simulink model "Lidar_System_FullState_Apr19_2015_Triangle"  (Simulink 7.3)
settings: Solver=FixedStepDiscrete  StartTime=0.0  StopTime=inf  FixedStep=0.1  MaxStep=0.2  RelTol=1e-3
undefined symbols (not defined in the file): strel
libraries: dspmtrx3 x9, simulink x7, vipstatistics x3, vipmorphops x3, dspstat3 x3, dspindex x1
(part 1 of 2)
settings Model: Creator=gclayton  LastModifiedBy=wildcat
settings DebuggingCC: InheritedTsInSrcMsg=none
settings RTWCC: SystemTargetFile=rlnx.tlc  GenCodeOnly=on  TemplateMakefile=rlnx_ubuntu.tmf  Description=Linux Real-Time Target  ProcessScript=rlnx_make_rtw_hook
settings RTWCC: CustomInclude=|
  | /usr/local/include/opencv/
  | /usr/local/include/
settings CodeAppCC: GenerateComments=off  SimulinkBlockComments=off
settings STFCustomTargetCC: ModelReferenceCompliant=off  MatFileLogging=on  SystemTargetFile=rlnx.tlc
settings GRTTargetCC: ModelReferenceCompliant=off  ParMdlRefBuildCompliant=off  CompOptLevelCompliant=off
settings CustomProperty: DataType=string  Value="-lm -ldl /usr/local/lib/libopencv_highgui.so.2.4 /usr/local/lib/libopencv_core.so.2.4 /usr/local/lib/libopencv_imgproc.so.2.4  -lc_urg -lc_urg_connection -lc_urg_system -lphidget21 -llcm"
settings EnumStrPairs: String=PC

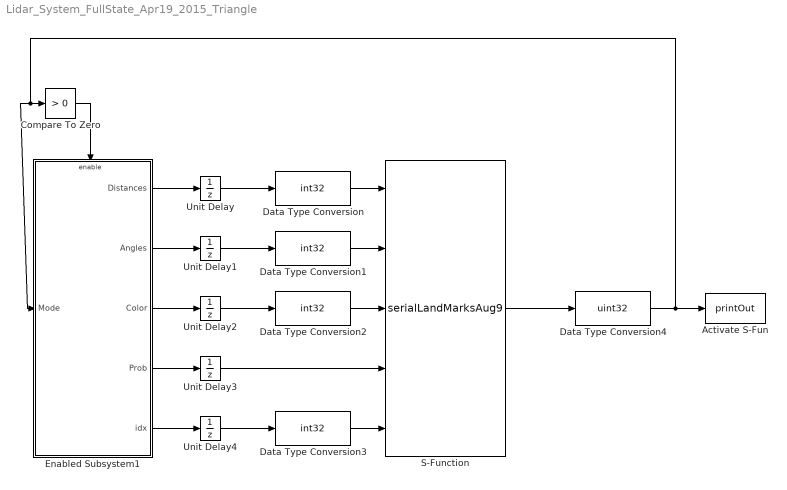
== system Lidar_System_FullState_Apr19_2015_Triangle ==
  Activate S-Fun : S-Function  FunctionName=printOut  EnableBusSupport=off
  Compare To Zero : simulink/Logic and Bit Operations/Compare To Zero  SystemSampleTime=-1  relop=>  LogicOutDataTypeMode=uint8  ZeroCross=off
  Data Type Conversion{,1..3} (4 alike) : DataTypeConversion  OutDataTypeMode=int32  OutDataType=fixdt(1, 16)  OutScaling=2^0  OutDataTypeStr=int32
  Data Type Conversion4 : DataTypeConversion  OutDataTypeMode=uint32  OutDataType=fixdt(1, 16)  OutScaling=2^0  OutDataTypeStr=uint32
  Enabled Subsystem1 : Subsystem  TreatAsAtomicUnit=on
  S-Function : S-Function  FunctionName=serialLandMarksAug9  EnableBusSupport=off
  Unit Delay : UnitDelay  X0=zeros(1,12)  SampleTime=-1
  Unit Delay1 : UnitDelay  X0=zeros(1,12)  SampleTime=-1
  Unit Delay2 : UnitDelay  X0=zeros(4,1)  SampleTime=-1
  Unit Delay3 : UnitDelay  X0=zeros(4,1)  SampleTime=-1
  Unit Delay4 : UnitDelay  X0=zeros(4,1)  SampleTime=-1
  wires:
  Compare To Zero/1 -> Enabled Subsystem1/Enable
  Data Type Conversion4/1 -> Activate S-Fun/1, Compare To Zero/1, Enabled Subsystem1/1(Mode)
  S-Function/1 -> Data Type Conversion4/1
  Enabled Subsystem1/2(Angles) -> Unit Delay1/1
  Enabled Subsystem1/1(Distances) -> Unit Delay/1
  Enabled Subsystem1/3(Color) -> Unit Delay2/1
  Enabled Subsystem1/4(Prob) -> Unit Delay3/1
  Enabled Subsystem1/5(idx) -> Unit Delay4/1
  Unit Delay/1 -> Data Type Conversion/1
  Unit Delay1/1 -> Data Type Conversion1/1
  Unit Delay2/1 -> Data Type Conversion2/1
  Unit Delay4/1 -> Data Type Conversion3/1
  Data Type Conversion/1 -> S-Function/1
  Data Type Conversion1/1 -> S-Function/2
  Data Type Conversion2/1 -> S-Function/3
  Unit Delay3/1 -> S-Function/4
  Data Type Conversion3/1 -> S-Function/5

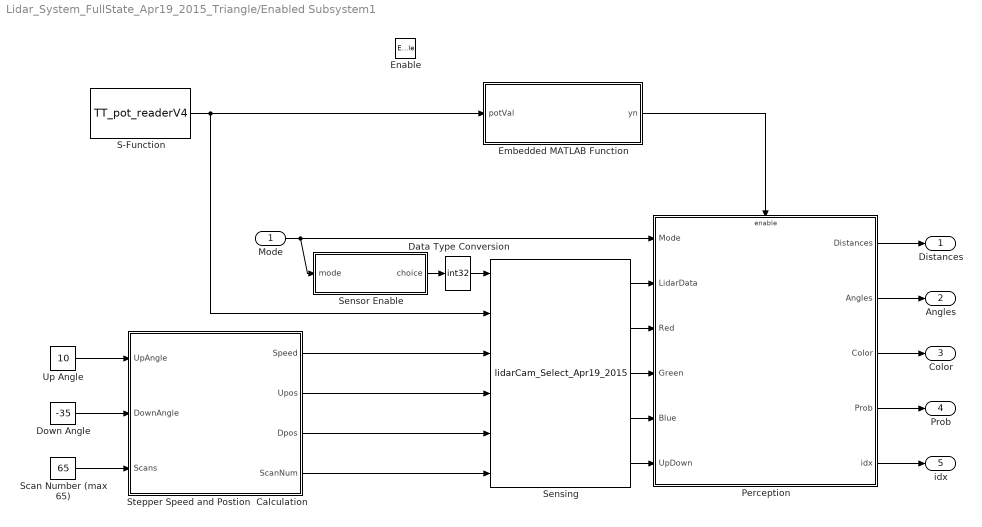
== system Lidar_System_FullState_Apr19_2015_Triangle/Enabled Subsystem1 ==
  Mode : Inport  OutDataType=fixdt(1, 16)  OutScaling=2^0
  Enable : EnablePort
  Data Type Conversion : DataTypeConversion  OutDataTypeMode=int32  OutDataType=fixdt(1, 16)  OutScaling=2^0  OutDataTypeStr=int32
  Down Angle : Constant  Value=-35  OutDataType=fixdt(1, 16)  OutScaling=2^0
  Embedded MATLAB Function : Stateflow chart
  Perception : Subsystem  TreatAsAtomicUnit=on
  S-Function : S-Function  FunctionName=TT_pot_readerV4  EnableBusSupport=off
  Scan Number (max 65) : Constant  Value=65  OutDataType=fixdt(1, 16)  OutScaling=2^0
  Sensing : S-Function  FunctionName=lidarCam_Select_Apr19_2015  EnableBusSupport=off
  Sensor Enable : Stateflow chart
  Stepper Speed and Postion  Calculation : Stateflow chart
  Up Angle : Constant  Value=10  OutDataType=fixdt(1, 16)  OutScaling=2^0
  Distances : Outport  OutDataType=fixdt(1, 16)  OutScaling=2^0
  Angles : Outport  Port=2  OutDataType=fixdt(1, 16)  OutScaling=2^0
  Color : Outport  Port=3  OutDataType=fixdt(1, 16)  OutScaling=2^0
  Prob : Outport  Port=4  OutDataType=fixdt(1, 16)  OutScaling=2^0
  idx : Outport  Port=5  OutDataType=fixdt(1, 16)  OutScaling=2^0
  wires:
  Embedded MATLAB Function/1(yn) -> Perception/Enable
  Sensing/1 -> Perception/2(LidarData)
  Sensing/5 -> Perception/6(UpDown)
  Sensing/2 -> Perception/3(Red)
  Sensing/3 -> Perception/4(Green)
  Sensing/4 -> Perception/5(Blue)
  Mode/1 -> Perception/1(Mode), Sensor Enable/1(mode)
  Down Angle/1 -> Stepper Speed and Postion  Calculation/2(DownAngle)
  Up Angle/1 -> Stepper Speed and Postion  Calculation/1(UpAngle)
  Scan Number (max 65)/1 -> Stepper Speed and Postion  Calculation/3(Scans)
  Stepper Speed and Postion  Calculation/1(Speed) -> Sensing/3
  Stepper Speed and Postion  Calculation/2(Upos) -> Sensing/4
  Stepper Speed and Postion  Calculation/3(Dpos) -> Sensing/5
  Stepper Speed and Postion  Calculation/4(ScanNum) -> Sensing/6
  S-Function/1 -> Embedded MATLAB Function/1(potVal), Sensing/2
  Sensor Enable/1(choice) -> Data Type Conversion/1
  Data Type Conversion/1 -> Sensing/1
  Perception/1(Distances) -> Distances/1
  Perception/2(Angles) -> Angles/1
  Perception/3(Color) -> Color/1
  Perception/4(Prob) -> Prob/1
  Perception/5(idx) -> idx/1

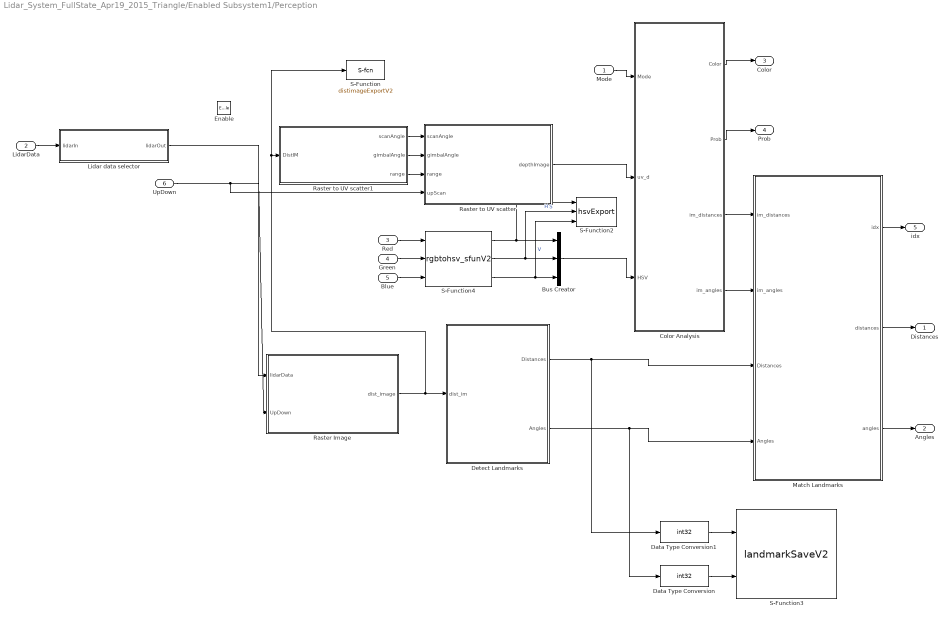
== system Lidar_System_FullState_Apr19_2015_Triangle/Enabled Subsystem1/Perception ==
  Mode : Inport  OutDataType=fixdt(1, 16)  OutScaling=2^0
  LidarData : Inport  Port=2  OutDataType=fixdt(1, 16)  OutScaling=2^0
  Red : Inport  Port=3  OutDataType=fixdt(1, 16)  OutScaling=2^0
  Green : Inport  Port=4  OutDataType=fixdt(1, 16)  OutScaling=2^0
  Blue : Inport  Port=5  OutDataType=fixdt(1, 16)  OutScaling=2^0
  UpDown : Inport  Port=6  OutDataType=fixdt(1, 16)  OutScaling=2^0
  Enable : EnablePort
  Bus Creator : BusCreator  Inputs=3
  Color Analysis : Subsystem
  Data Type Conversion : DataTypeConversion  OutDataTypeMode=int32  OutDataType=fixdt(1, 16)  OutScaling=2^0  OutDataTypeStr=int32
  Data Type Conversion1 : DataTypeConversion  OutDataTypeMode=int32  OutDataType=fixdt(1, 16)  OutScaling=2^0  OutDataTypeStr=int32
  Detect Landmarks : Subsystem
  Lidar data selector : Stateflow chart
  Match Landmarks : Stateflow chart
  Raster Image : Stateflow chart
  Raster to UV scatter : Stateflow chart
  Raster to UV scatter1 : Stateflow chart
  S-Function : S-Function  FunctionName=distimageExportV2  EnableBusSupport=off
  S-Function2 : S-Function  FunctionName=hsvExport  EnableBusSupport=off
  S-Function3 : S-Function  FunctionName=landmarkSaveV2  EnableBusSupport=off
  S-Function4 : S-Function  FunctionName=rgbtohsv_sfunV2  EnableBusSupport=off
  Distances : Outport  OutDataType=fixdt(1, 16)  OutScaling=2^0
  Angles : Outport  Port=2  OutDataType=fixdt(1, 16)  OutScaling=2^0
  Color : Outport  Port=3  OutDataType=fixdt(1, 16)  OutScaling=2^0
  Prob : Outport  Port=4  OutDataType=fixdt(1, 16)  OutScaling=2^0
  idx : Outport  Port=5  OutDataType=fixdt(1, 16)  OutScaling=2^0
  wires:
  Lidar data selector/1(lidarOut) -> Raster Image/1(lidarData)
  UpDown/1 -> Raster Image/2(UpDown), Raster to UV scatter/4(upScan)
  Red/1 -> S-Function4/1
  Green/1 -> S-Function4/2
  Blue/1 -> S-Function4/3
  LidarData/1 -> Lidar data selector/1(lidarIn)
  S-Function4/1 -> Bus Creator/1, S-Function2/1  "H"
  S-Function4/2 -> Bus Creator/2, S-Function2/2  "S"
  S-Function4/3 -> Bus Creator/3, S-Function2/3  "V"
  Bus Creator/1 -> Color Analysis/3(HSV)
  Raster to UV scatter/1(depthImage) -> Color Analysis/2(uv_d)
  Mode/1 -> Color Analysis/1(Mode)
  Color Analysis/2(Prob) -> Prob/1
  Color Analysis/1(Color) -> Color/1
  Color Analysis/3(im_distances) -> Match Landmarks/1(im_distances)
  Color Analysis/4(im_angles) -> Match Landmarks/2(im_angles)
  Detect Landmarks/1(Distances) -> Match Landmarks/3(Distances), Data Type Conversion1/1
  Detect Landmarks/2(Angles) -> Match Landmarks/4(Angles), Data Type Conversion/1
  Raster Image/1(dist_image) -> Detect Landmarks/1(dist_im), Raster to UV scatter1/1(DistIM), S-Function/1
  Raster to UV scatter1/1(scanAngle) -> Raster to UV scatter/1(scanAngle)
  Raster to UV scatter1/2(gimbalAngle) -> Raster to UV scatter/2(gimbalAngle)
  Raster to UV scatter1/3(range) -> Raster to UV scatter/3(range)
  Match Landmarks/1(idx) -> idx/1
  Match Landmarks/2(distances) -> Distances/1
  Match Landmarks/3(angles) -> Angles/1
  Data Type Conversion/1 -> S-Function3/2
  Data Type Conversion1/1 -> S-Function3/1

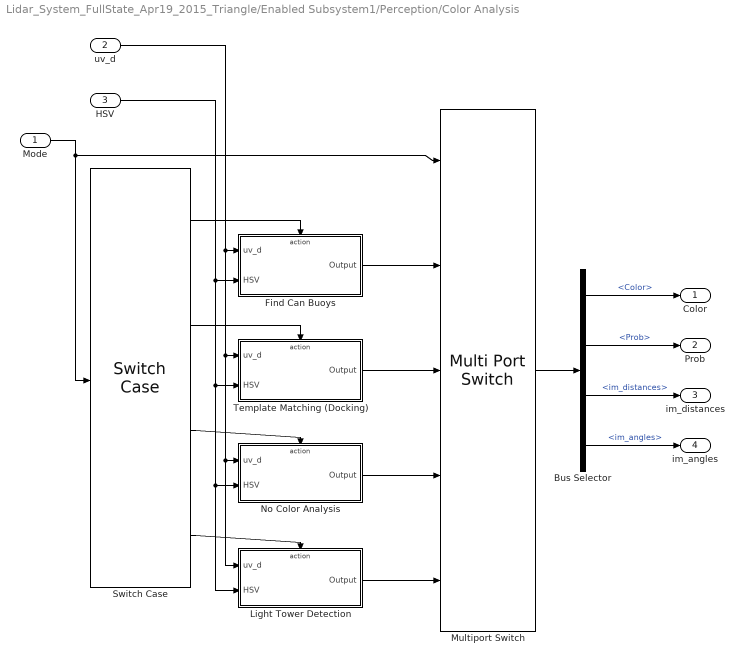
== system Lidar_System_FullState_Apr19_2015_Triangle/Enabled Subsystem1/Perception/Color Analysis ==
  Mode : Inport  OutDataType=fixdt(1, 16)  OutScaling=2^0
  uv_d : Inport  Port=2  OutDataType=fixdt(1, 16)  OutScaling=2^0
  HSV : Inport  Port=3  OutDataType=fixdt(1, 16)  OutScaling=2^0
  Bus Selector : BusSelector  OutputSignals=Color,Prob,im_distances,im_angles
  Find Can Buoys : Subsystem  TreatAsAtomicUnit=on
  Light Tower Detection : Subsystem  TreatAsAtomicUnit=on
  Multiport Switch : MultiPortSwitch  Inputs=4  OutDataType=fixdt(1, 16)  OutScaling=2^0
  No Color Analysis : Subsystem  TreatAsAtomicUnit=on
  Switch Case : SwitchCase  CaseConditions={1,2,3}
  Template Matching (Docking) : Subsystem  TreatAsAtomicUnit=on
  Color : Outport  OutDataType=fixdt(1, 16)  OutScaling=2^0
  Prob : Outport  Port=2  OutDataType=fixdt(1, 16)  OutScaling=2^0
  im_distances : Outport  Port=3  OutDataType=fixdt(1, 16)  OutScaling=2^0
  im_angles : Outport  Port=4  OutDataType=fixdt(1, 16)  OutScaling=2^0
  wires:
  Switch Case/1 -> Find Can Buoys/Action
  Mode/1 -> Switch Case/1, Multiport Switch/1
  Switch Case/2 -> Template Matching (Docking)/Action
  Switch Case/3 -> No Color Analysis/Action
  Switch Case/4 -> Light Tower Detection/Action
  Find Can Buoys/1(Output) -> Multiport Switch/2
  No Color Analysis/1(Output) -> Multiport Switch/4
  Light Tower Detection/1(Output) -> Multiport Switch/5
  uv_d/1 -> Light Tower Detection/1(uv_d), No Color Analysis/1(uv_d), Template Matching (Docking)/1(uv_d), Find Can Buoys/1(uv_d)
  HSV/1 -> Light Tower Detection/2(HSV), No Color Analysis/2(HSV), Template Matching (Docking)/2(HSV), Find Can Buoys/2(HSV)
  Template Matching (Docking)/1(Output) -> Multiport Switch/3
  Multiport Switch/1 -> Bus Selector/1
  Bus Selector/1 -> Color/1  "<Color>"
  Bus Selector/2 -> Prob/1  "<Prob>"
  Bus Selector/3 -> im_distances/1  "<im_distances>"
  Bus Selector/4 -> im_angles/1  "<im_angles>"

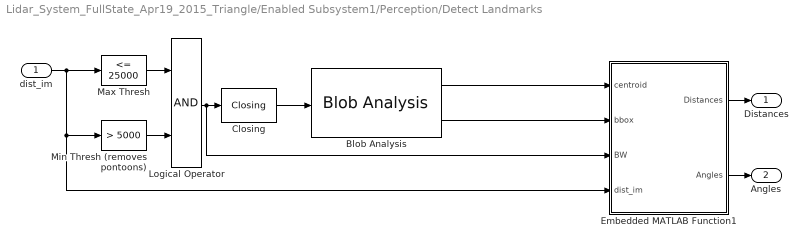
== system Lidar_System_FullState_Apr19_2015_Triangle/Enabled Subsystem1/Perception/Detect Landmarks ==
  dist_im : Inport  OutDataType=fixdt(1, 16)  OutScaling=2^0
  Blob Analysis : vipstatistics/Blob Analysis  DialogController=vipDDGCreate  DialogControllerArgs=DataTag5  area=off  centroid=on  bBox=on  majorAxis=off  minorAxis=off  angle=off  eccentricity=off  equivDiameterSq=off  extent=off  perimeter=off  maxBlobs=12  warnIfNumBlobsExceeded=on  isCount=off  useMinArea=on  minArea=30  useMaxArea=off  maxArea=intmax('uint32')  excludeBorderBlob=on  outDT=double  isOutVarDim=off  isFill=on  fillValues=-1  conn=8  isLabel=off  outputMode=Binary point scaling  outputWordLength=32  outputFracLength=16  firstCoeffMode=Binary point scaling  firstCoeffWordLength=16  firstCoeffFracLength=14  secondCoeffMode=Binary point scaling  secondCoeffWordLength=32  secondCoeffFracLength=16  accumMode=Binary point scaling  accumWordLength=32  accumFracLength=0  prodOutputMode=Binary point scaling  prodOutputWordLength=32  prodOutputFracLength=16  roundingMode=Floor  overflowMode=off
  Closing : vipmorphops/Closing  nhoodsrc=Specify via dialog  strel=strel('rectangle',[5 7])
  Embedded MATLAB Function1 : Stateflow chart
  Logical Operator : Logic  AllPortsSameDT=off  OutDataTypeMode=boolean  LogicDataType=fixdt(0, 8)  OutDataTypeStr=boolean
  Max Thresh : simulink/Logic and Bit Operations/Compare To Constant  SystemSampleTime=-1  relop=<=  const=25000  LogicOutDataTypeMode=boolean  ZeroCross=off
  Min Thresh (removes pontoons) : simulink/Logic and Bit Operations/Compare To Constant  SystemSampleTime=-1  relop=>  const=5000  LogicOutDataTypeMode=boolean  ZeroCross=off
  Distances : Outport  OutDataType=fixdt(1, 16)  OutScaling=2^0
  Angles : Outport  Port=2  OutDataType=fixdt(1, 16)  OutScaling=2^0
  wires:
  Max Thresh/1 -> Logical Operator/1
  Min Thresh (removes pontoons)/1 -> Logical Operator/2
  dist_im/1 -> Max Thresh/1, Min Thresh (removes pontoons)/1, Embedded MATLAB Function1/4(dist_im)
  Embedded MATLAB Function1/1(Distances) -> Distances/1
  Embedded MATLAB Function1/2(Angles) -> Angles/1
  Logical Operator/1 -> Closing/1, Embedded MATLAB Function1/3(BW)
  Closing/1 -> Blob Analysis/1
  Blob Analysis/1 -> Embedded MATLAB Function1/1(centroid)
  Blob Analysis/2 -> Embedded MATLAB Function1/2(bbox)

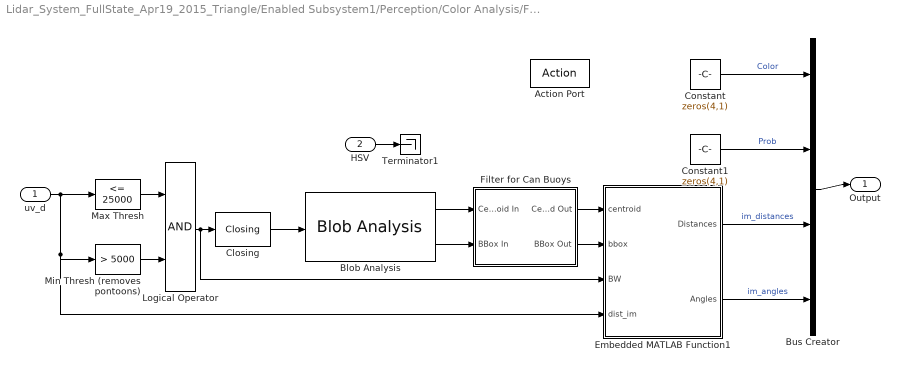
== system Lidar_System_FullState_Apr19_2015_Triangle/Enabled Subsystem1/Perception/Color Analysis/Find Can Buoys ==
  uv_d : Inport  OutDataType=fixdt(1, 16)  OutScaling=2^0
  HSV : Inport  Port=2  OutDataType=fixdt(1, 16)  OutScaling=2^0
  Action Port : ActionPort  ActionType=case
  Blob Analysis : vipstatistics/Blob Analysis  DialogController=vipDDGCreate  DialogControllerArgs=DataTag0  area=off  centroid=on  bBox=on  majorAxis=off  minorAxis=off  angle=off  eccentricity=off  equivDiameterSq=off  extent=off  perimeter=off  maxBlobs=12  warnIfNumBlobsExceeded=on  isCount=off  useMinArea=on  minArea=30  useMaxArea=off  maxArea=intmax('uint32')  excludeBorderBlob=on  outDT=double  isOutVarDim=off  isFill=on  fillValues=-1  conn=8  isLabel=off  outputMode=Binary point scaling  outputWordLength=32  outputFracLength=16  firstCoeffMode=Binary point scaling  firstCoeffWordLength=16  firstCoeffFracLength=14  secondCoeffMode=Binary point scaling  secondCoeffWordLength=32  secondCoeffFracLength=16  accumMode=Binary point scaling  accumWordLength=32  accumFracLength=0  prodOutputMode=Binary point scaling  prodOutputWordLength=32  prodOutputFracLength=16  roundingMode=Floor  overflowMode=off
  Bus Creator : BusCreator
  Closing : vipmorphops/Closing  nhoodsrc=Specify via dialog  strel=strel('rectangle',[5 7])
  Constant : Constant  Value=zeros(4,1)  OutDataType=fixdt(1, 16)  OutScaling=2^0
  Constant1 : Constant  Value=zeros(4,1)  OutDataType=fixdt(1, 16)  OutScaling=2^0
  Embedded MATLAB Function1 : Stateflow chart
  Filter for Can Buoys : Subsystem
  Logical Operator : Logic  AllPortsSameDT=off  OutDataTypeMode=boolean  LogicDataType=fixdt(0, 8)  OutDataTypeStr=boolean
  Max Thresh : simulink/Logic and Bit Operations/Compare To Constant  SystemSampleTime=-1  relop=<=  const=25000  LogicOutDataTypeMode=boolean  ZeroCross=off
  Min Thresh (removes pontoons) : simulink/Logic and Bit Operations/Compare To Constant  SystemSampleTime=-1  relop=>  const=5000  LogicOutDataTypeMode=boolean  ZeroCross=off
  Terminator1 : Terminator
  Output : Outport  OutDataType=fixdt(1, 16)  OutScaling=2^0
  wires:
  Constant/1 -> Bus Creator/1  "Color"
  Constant1/1 -> Bus Creator/2  "Prob"
  Embedded MATLAB Function1/1(Distances) -> Bus Creator/3  "im_distances"
  Embedded MATLAB Function1/2(Angles) -> Bus Creator/4  "im_angles"
  Bus Creator/1 -> Output/1
  HSV/1 -> Terminator1/1
  Max Thresh/1 -> Logical Operator/1
  Min Thresh (removes pontoons)/1 -> Logical Operator/2
  Logical Operator/1 -> Closing/1, Embedded MATLAB Function1/3(BW)
  Closing/1 -> Blob Analysis/1
  uv_d/1 -> Max Thresh/1, Min Thresh (removes pontoons)/1, Embedded MATLAB Function1/4(dist_im)
  Blob Analysis/1 -> Filter for Can Buoys/1(Centroid In)
  Blob Analysis/2 -> Filter for Can Buoys/2(BBox In)
  Filter for Can Buoys/1(Centroid Out) -> Embedded MATLAB Function1/1(centroid)
  Filter for Can Buoys/2(BBox Out) -> Embedded MATLAB Function1/2(bbox)

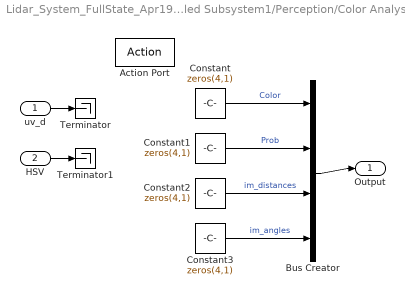
== system Lidar_System_FullState_Apr19_2015_Triangle/Enabled Subsystem1/Perception/Color Analysis/Light Tower Detection ==
  uv_d : Inport  OutDataType=fixdt(1, 16)  OutScaling=2^0
  HSV : Inport  Port=2  OutDataType=fixdt(1, 16)  OutScaling=2^0
  Action Port : ActionPort  ActionType=default
  Bus Creator : BusCreator
  Constant{,1..3} (4 alike) : Constant  Value=zeros(4,1)  OutDataType=fixdt(1, 16)  OutScaling=2^0
  Terminator : Terminator
  Terminator1 : Terminator
  Output : Outport  OutDataType=fixdt(1, 16)  OutScaling=2^0
  wires:
  uv_d/1 -> Terminator/1
  HSV/1 -> Terminator1/1
  Constant/1 -> Bus Creator/1  "Color"
  Constant1/1 -> Bus Creator/2  "Prob"
  Constant2/1 -> Bus Creator/3  "im_distances"
  Constant3/1 -> Bus Creator/4  "im_angles"
  Bus Creator/1 -> Output/1

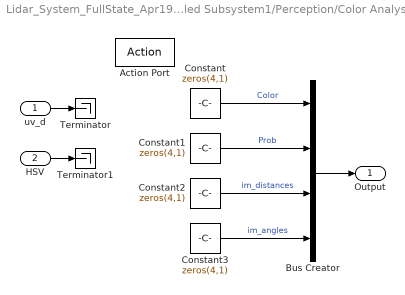
== system Lidar_System_FullState_Apr19_2015_Triangle/Enabled Subsystem1/Perception/Color Analysis/No Color Analysis ==
  uv_d : Inport  OutDataType=fixdt(1, 16)  OutScaling=2^0
  HSV : Inport  Port=2  OutDataType=fixdt(1, 16)  OutScaling=2^0
  Action Port : ActionPort  ActionType=case
  Bus Creator : BusCreator
  Constant{,1..3} (4 alike) : Constant  Value=zeros(4,1)  OutDataType=fixdt(1, 16)  OutScaling=2^0
  Terminator : Terminator
  Terminator1 : Terminator
  Output : Outport  OutDataType=fixdt(1, 16)  OutScaling=2^0
  wires:
  Constant/1 -> Bus Creator/1  "Color"
  Constant1/1 -> Bus Creator/2  "Prob"
  Constant2/1 -> Bus Creator/3  "im_distances"
  Constant3/1 -> Bus Creator/4  "im_angles"
  Bus Creator/1 -> Output/1
  HSV/1 -> Terminator1/1
  uv_d/1 -> Terminator/1

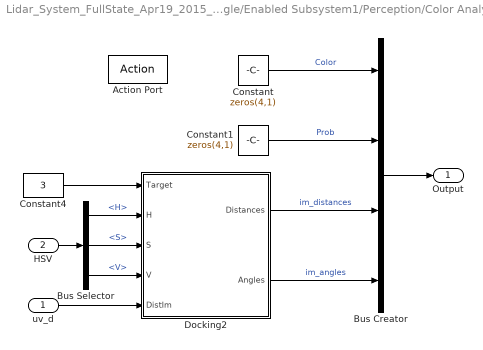
== system Lidar_System_FullState_Apr19_2015_Triangle/Enabled Subsystem1/Perception/Color Analysis/Template Matching (Docking) ==
  uv_d : Inport  OutDataType=fixdt(1, 16)  OutScaling=2^0
  HSV : Inport  Port=2  OutDataType=fixdt(1, 16)  OutScaling=2^0
  Action Port : ActionPort  ActionType=case
  Bus Creator : BusCreator
  Bus Selector : BusSelector  OutputSignals=H,S,V
  Constant : Constant  Value=zeros(4,1)  OutDataType=fixdt(1, 16)  OutScaling=2^0
  Constant1 : Constant  Value=zeros(4,1)  OutDataType=fixdt(1, 16)  OutScaling=2^0
  Constant4 : Constant  Value=3  OutDataType=fixdt(1, 16)  OutScaling=2^0
  Docking2 : Subsystem
  Output : Outport  OutDataType=fixdt(1, 16)  OutScaling=2^0
  wires:
  Constant/1 -> Bus Creator/1  "Color"
  Constant1/1 -> Bus Creator/2  "Prob"
  Docking2/1(Distances) -> Bus Creator/3  "im_distances"
  Docking2/2(Angles) -> Bus Creator/4  "im_angles"
  Bus Creator/1 -> Output/1
  Constant4/1 -> Docking2/1(Target)
  Bus Selector/1 -> Docking2/2(H)  "<H>"
  Bus Selector/2 -> Docking2/3(S)  "<S>"
  Bus Selector/3 -> Docking2/4(V)  "<V>"
  HSV/1 -> Bus Selector/1
  uv_d/1 -> Docking2/5(DistIm)

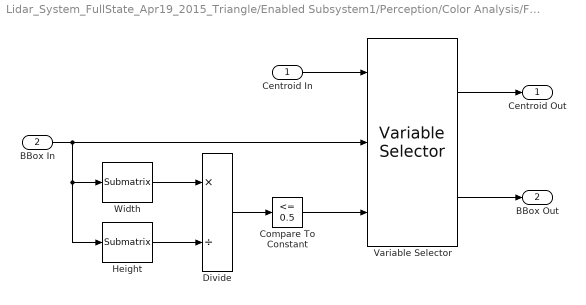
== system Lidar_System_FullState_Apr19_2015_Triangle/Enabled Subsystem1/Perception/Color Analysis/Find Can Buoys/Filter for Can Buoys ==
  Centroid In : Inport  OutDataType=fixdt(1, 16)  OutScaling=2^0
  BBox In : Inport  Port=2  OutDataType=fixdt(1, 16)  OutScaling=2^0
  Compare To Constant : simulink/Logic and Bit Operations/Compare To Constant  SystemSampleTime=-1  relop=<=  const=0.5  LogicOutDataTypeMode=uint8  ZeroCross=off
  Divide : Product  Inputs=*/  OutDataType=fixdt(1, 16)  OutScaling=2^-10
  Height : dspmtrx3/Submatrix  RowSpan=One row  RowStartMode=Index  RowStartIndex=4  RowEndMode=Last  RowEndIndex=1  ColSpan=All columns  ColStartMode=First  ColStartIndex=1  ColEndMode=Last  ColEndIndex=1
  Variable Selector : dspindex/Variable Selector  NumInputs=2  rowsOrCols=Columns  IdxMode=Variable  Elements=[1 3]  ZerOneIdxMode=Zero-based  errmode=Clip Index  FillMode=on  FillValues=-1
  Width : dspmtrx3/Submatrix  RowSpan=One row  RowStartMode=Index  RowStartIndex=3  RowEndMode=Last  RowEndIndex=1  ColSpan=All columns  ColStartMode=First  ColStartIndex=1  ColEndMode=Last  ColEndIndex=1
  Centroid Out : Outport  OutDataType=fixdt(1, 16)  OutScaling=2^0
  BBox Out : Outport  Port=2  OutDataType=fixdt(1, 16)  OutScaling=2^0
  wires:
  Centroid In/1 -> Variable Selector/1
  BBox In/1 -> Width/1, Height/1, Variable Selector/2
  Width/1 -> Divide/1
  Height/1 -> Divide/2
  Divide/1 -> Compare To Constant/1
  Compare To Constant/1 -> Variable Selector/3
  Variable Selector/2 -> BBox Out/1
  Variable Selector/1 -> Centroid Out/1

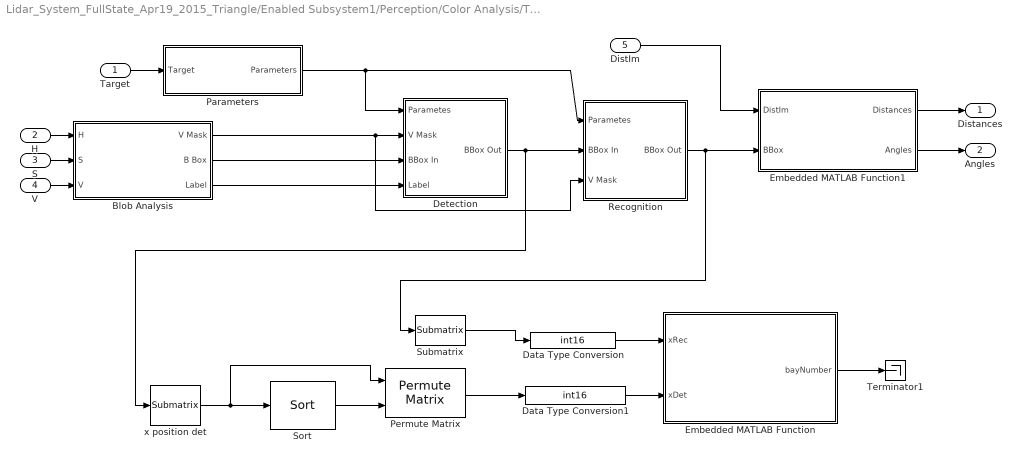
== system Lidar_System_FullState_Apr19_2015_Triangle/Enabled Subsystem1/Perception/Color Analysis/Template Matching (Docking)/Docking2 ==
  Target : Inport
  H : Inport  Port=2
  S : Inport  Port=3
  V : Inport  Port=4
  DistIm : Inport  Port=5
  Blob Analysis : Subsystem
  Data Type Conversion : DataTypeConversion  OutDataTypeMode=int16  OutDataType=fixdt(1, 16)  OutScaling=2^0  OutDataTypeStr=int16
  Data Type Conversion1 : DataTypeConversion  OutDataTypeMode=int16  OutDataType=fixdt(1, 16)  OutScaling=2^0  OutDataTypeStr=int16
  Detection : Subsystem
  Embedded MATLAB Function : Stateflow chart
  Embedded MATLAB Function1 : Stateflow chart
  Parameters : Subsystem
  Permute Matrix : dspmtrx3/Permute Matrix  mode=Rows  ZeroOneIdxMode=One-based  errmode=Clip index  checkDims=off
  Recognition : Subsystem
  Sort : dspstat3/Sort  DialogController=dspDDGCreate  DialogControllerArgs=DataTag4  otype=Index  dir=Ascending  sortAlg=Quick sort  roundingMode=Floor  overflowMode=off
  Submatrix : dspmtrx3/Submatrix  RowSpan=Range of rows  RowStartMode=First  RowStartIndex=1  RowEndMode=Last  RowEndIndex=1  ColSpan=One column  ColStartMode=First  ColStartIndex=1  ColEndMode=Last  ColEndIndex=1
  Terminator1 : Terminator
  x position det : dspmtrx3/Submatrix  RowSpan=Range of rows  RowStartMode=First  RowStartIndex=1  RowEndMode=Last  RowEndIndex=1  ColSpan=One column  ColStartMode=First  ColStartIndex=1  ColEndMode=Last  ColEndIndex=1
  Distances : Outport
  Angles : Outport  Port=2
  wires:
  Parameters/1(Parameters) -> Detection/1(Parametes), Recognition/1(Parametes)
  Blob Analysis/1(V Mask) -> Detection/2(V Mask), Recognition/3(V Mask)
  Blob Analysis/2(B Box) -> Detection/3(BBox In)
  Blob Analysis/3(Label) -> Detection/4(Label)
  Detection/1(BBox Out) -> Recognition/2(BBox In), x position det/1
  x position det/1 -> Sort/1, Permute Matrix/1
  Sort/1 -> Permute Matrix/2
  Submatrix/1 -> Data Type Conversion/1
  Permute Matrix/1 -> Data Type Conversion1/1
  Data Type Conversion/1 -> Embedded MATLAB Function/1(xRec)
  Data Type Conversion1/1 -> Embedded MATLAB Function/2(xDet)
  Recognition/1(BBox Out) -> Submatrix/1, Embedded MATLAB Function1/2(BBox)
  Embedded MATLAB Function/1(bayNumber) -> Terminator1/1
  DistIm/1 -> Embedded MATLAB Function1/1(DistIm)
  Embedded MATLAB Function1/1(Distances) -> Distances/1
  H/1 -> Blob Analysis/1(H)
  S/1 -> Blob Analysis/2(S)
  V/1 -> Blob Analysis/3(V)
  Target/1 -> Parameters/1(Target)
  Embedded MATLAB Function1/2(Angles) -> Angles/1

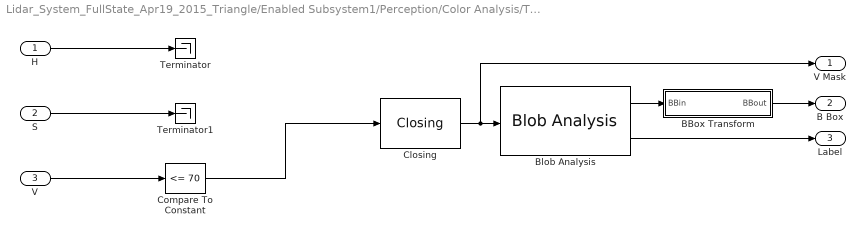
== system Lidar_System_FullState_Apr19_2015_Triangle/Enabled Subsystem1/Perception/Color Analysis/Template Matching (Docking)/Docking2/Blob Analysis ==
  H : Inport  OutDataType=fixdt(1, 16)  OutScaling=2^0
  S : Inport  Port=2  OutDataType=fixdt(1, 16)  OutScaling=2^0
  V : Inport  Port=3  OutDataType=fixdt(1, 16)  OutScaling=2^0
  BBox Transform : Stateflow chart
  Blob Analysis : vipstatistics/Blob Analysis  DialogController=vipDDGCreate  DialogControllerArgs=DataTag1  area=off  centroid=off  bBox=on  majorAxis=off  minorAxis=off  angle=off  eccentricity=off  equivDiameterSq=off  extent=off  perimeter=off  maxBlobs=10  warnIfNumBlobsExceeded=on  isCount=off  useMinArea=on  minArea=400  useMaxArea=off  maxArea=intmax('uint32')  excludeBorderBlob=on  outDT=double  isOutVarDim=off  isFill=on  fillValues=-1  conn=8  isLabel=on  outputMode=Binary point scaling  outputWordLength=32  outputFracLength=16  firstCoeffMode=Binary point scaling  firstCoeffWordLength=16  firstCoeffFracLength=14  secondCoeffMode=Binary point scaling  secondCoeffWordLength=32  secondCoeffFracLength=16  accumMode=Binary point scaling  accumWordLength=32  accumFracLength=0  prodOutputMode=Binary point scaling  prodOutputWordLength=32  prodOutputFracLength=16  roundingMode=Floor  overflowMode=off
  Closing : vipmorphops/Closing  nhoodsrc=Specify via dialog  strel=strel('disk',1,8)
  Compare To Constant : simulink/Logic and Bit Operations/Compare To Constant  SystemSampleTime=-1  relop=<=  const=70  LogicOutDataTypeMode=boolean  ZeroCross=off
  Terminator : Terminator
  Terminator1 : Terminator
  V Mask : Outport  OutDataType=fixdt(1, 16)  OutScaling=2^0
  B Box : Outport  Port=2  OutDataType=fixdt(1, 16)  OutScaling=2^0
  Label : Outport  Port=3  OutDataType=fixdt(1, 16)  OutScaling=2^0
  wires:
  Blob Analysis/2 -> Label/1
  Blob Analysis/1 -> BBox Transform/1(BBin)
  Closing/1 -> Blob Analysis/1, V Mask/1
  BBox Transform/1(BBout) -> B Box/1
  V/1 -> Compare To Constant/1
  S/1 -> Terminator1/1
  H/1 -> Terminator/1
  Compare To Constant/1 -> Closing/1

== system Lidar_System_FullState_Apr19_2015_Triangle/Enabled Subsystem1/Perception/Color Analysis/Template Matching (Docking)/Docking2/Detection ==
  Parametes : Inport  OutDataType=fixdt(1, 16)  OutScaling=2^0
  V Mask : Inport  Port=2  OutDataType=fixdt(1, 16)  OutScaling=2^0
  BBox In : Inport  Port=3  OutDataType=fixdt(1, 16)  OutScaling=2^0
  Label : Inport  Port=4  OutDataType=fixdt(1, 16)  OutScaling=2^0
  Bus Selector : BusSelector  OutputSignals=Templates.Cruciform,Templates.Circle,Templates.Triangle,White Pix Count,Threshold
  Detection : Stateflow chart
  Subsystem : Subsystem
  BBox Out : Outport  OutDataType=fixdt(1, 16)  OutScaling=2^0
  wires:
  Parametes/1 -> Bus Selector/1
  Bus Selector/1 -> Detection/1(cruciform)  "<Cruciform>"
  Bus Selector/2 -> Detection/2(circle)  "<Circle>"
  Bus Selector/3 -> Detection/3(triangle)  "<Triangle>"
  Bus Selector/4 -> Detection/4(whitePixCount)  "<White Pix Count>"
  Bus Selector/5 -> Detection/5(threshold)  "<Threshold>"
  V Mask/1 -> Detection/6(V_mask)
  BBox In/1 -> Detection/7(bbox_in)
  Label/1 -> Detection/8(label)
  Detection/2(rtnRatioDiff) -> Subsystem/2(Idx)
  Detection/1(bbox_out) -> Subsystem/1(BBox in)
  Subsystem/1(BBox out) -> BBox Out/1

== system Lidar_System_FullState_Apr19_2015_Triangle/Enabled Subsystem1/Perception/Color Analysis/Template Matching (Docking)/Docking2/Parameters ==
  Target : Inport
  Bus Creator : BusCreator
  Ratio Difference Threshold : Constant  Value=0.6  OutDataType=fixdt(1, 16)  OutScaling=2^0
  Templates : Subsystem
  White Pixel Count : Constant  Value="[144\t64\t180]"  OutDataType=fixdt(1, 16)  OutScaling=2^0
  Parameters : Outport  OutDataType=fixdt(1, 16)  OutScaling=2^0
  wires:
  Target/1 -> Bus Creator/1  "Target Template"
  Templates/1(Templates) -> Bus Creator/2  "Templates"
  White Pixel Count/1 -> Bus Creator/3  "White Pix Count"
  Ratio Difference Threshold/1 -> Bus Creator/4  "Threshold"
  Bus Creator/1 -> Parameters/1

== system Lidar_System_FullState_Apr19_2015_Triangle/Enabled Subsystem1/Perception/Color Analysis/Template Matching (Docking)/Docking2/Recognition ==
  Parametes : Inport  OutDataType=fixdt(1, 16)  OutScaling=2^0
  BBox In : Inport  Port=2  OutDataType=fixdt(1, 16)  OutScaling=2^0
  V Mask : Inport  Port=3  OutDataType=fixdt(1, 16)  OutScaling=2^0
  Bus Selector : BusSelector  OutputSignals=Target Template,Templates.Cruciform,Templates.Circle,Templates.Triangle,White Pix Count,Threshold
  Embedded MATLAB Function : Stateflow chart
  Subsystem : Subsystem
  BBox Out : Outport  OutDataType=fixdt(1, 16)  OutScaling=2^0
  wires:
  Subsystem/1(BBox out) -> BBox Out/1
  Parametes/1 -> Bus Selector/1
  Bus Selector/1 -> Embedded MATLAB Function/1(targetTemp)  "<Target Template>"
  Bus Selector/2 -> Embedded MATLAB Function/2(cruciform)  "<Cruciform>"
  Bus Selector/3 -> Embedded MATLAB Function/3(circle)  "<Circle>"
  Bus Selector/4 -> Embedded MATLAB Function/4(triangle)  "<Triangle>"
  Bus Selector/5 -> Embedded MATLAB Function/5(whitePixCount)  "<White Pix Count>"
  Bus Selector/6 -> Embedded MATLAB Function/6(threshold)  "<Threshold>"
  V Mask/1 -> Embedded MATLAB Function/7(V_mask)
  BBox In/1 -> Embedded MATLAB Function/8(bbox_in)
  Embedded MATLAB Function/1(bbox_out) -> Subsystem/1(BBox in)
  Embedded MATLAB Function/2(returnRatioDiff) -> Subsystem/2(Idx)

== system Lidar_System_FullState_Apr19_2015_Triangle/Enabled Subsystem1/Perception/Color Analysis/Template Matching (Docking)/Docking2/Detection/Subsystem ==
  BBox in : Inport  OutDataType=fixdt(1, 16)  OutScaling=2^0
  Idx : Inport  Port=2  OutDataType=fixdt(1, 16)  OutScaling=2^0
  Permute Matrix : dspmtrx3/Permute Matrix  mode=Rows  ZeroOneIdxMode=One-based  errmode=Clip index  checkDims=off
  Sort : dspstat3/Sort  DialogController=dspDDGCreate  DialogControllerArgs=DataTag2  otype=Index  dir=Ascending  sortAlg=Quick sort  roundingMode=Floor  overflowMode=off
  Submatrix : dspmtrx3/Submatrix  RowSpan=Range of rows  RowStartMode=First  RowStartIndex=1  RowEndMode=Index  RowEndIndex=3  ColSpan=Range of columns  ColStartMode=First  ColStartIndex=1  ColEndMode=Last  ColEndIndex=1
  BBox out : Outport  OutDataType=fixdt(1, 16)  OutScaling=2^0
  wires:
  Idx/1 -> Sort/1
  BBox in/1 -> Permute Matrix/1
  Sort/1 -> Permute Matrix/2
  Permute Matrix/1 -> Submatrix/1
  Submatrix/1 -> BBox out/1

== system Lidar_System_FullState_Apr19_2015_Triangle/Enabled Subsystem1/Perception/Color Analysis/Template Matching (Docking)/Docking2/Parameters/Templates ==
  Bus Creator : BusCreator  Inputs=3
  Circle : Constant  Value=|  OutDataType=fixdt(1, 16)  OutScaling=2^0
      | [1	1	1	1	1	1	0	0	0	0	0	0	0	1	1	1	1	1	1
      | 1	1	1	1	0	0	0	0	0	0	0	0	0	0	0	1	1	1	1
      | 1	1	0	0	0	0	0	0	0	0	0	0	0	0	0	0	0	1	1
      | 1	1	0	0	0	0	0	0	0	0	0	0	0	0	0	0	0	1	1
      | 1	0	0	0	0	0	0	0	0	0	0	0	0	0	0	0	0	0	1
      | 1	0	0	0	0	0	0	0	0	0	0	0	0	0	0	0	0	0	1
      | 0	0	0	0	0	0	0	0	0	0	0	0	0	0	0	0	0	0	0
      | 0	0	0	0	0	0	0	0	0	0	0	0	0	0	0	0	0	0	0
      | 0	0	0	0	0	0	0	0	0	0	0	0	0	0	0	0	0	0	0
      | 0	0	0	0	0	0	0	0	0	0	0	0	0	0	0	0	0	0	0
      | 0	0	0	0	0	0	0	0	0	0	0	0	0	0	0	0	0	0	0
      | 0	0	0	0	0	0	0	0	0	0	0	0	0	0	0	0	0	0	0
      | 0	0	0	0	0	0	0	0	0	0	0	0	0	0	0	0	0	0	0
      | 1	0	0	0	0	0	0	0	0	0	0	0	0	0	0	0	0	0	1
      | 1	0	0	0	0	0	0	0	0	0	0	0	0	0	0	0	0	0	1
      | 1	1	0	0	0	0	0	0	0	0	0	0	0	0	0	0	0	1	1
      | 1	1	0	0	0	0	0	0	0	0	0	0	0	0	0	0	0	1	1
      | 1	1	1	1	0	0	0	0	0	0	0	0	0	0	0	1	1	1	1
      | 1	1	1	1	1	1	0	0	0	0	0	0	0	1	1	1	1	1	1]
  Cruciform : Constant  Value=|  OutDataType=fixdt(1, 16)  OutScaling=2^0
      | [1	1	1	1	1	1	0	0	0	0	0	0	0	1	1	1	1	1	1
      | 1	1	1	1	1	1	0	0	0	0	0	0	0	1	1	1	1	1	1
      | 1	1	1	1	1	1	0	0	0	0	0	0	0	1	1	1	1	1	1
      | 1	1	1	1	1	1	0	0	0	0	0	0	0	1	1	1	1	1	1
      | 1	1	1	1	1	1	0	0	0	0	0	0	0	1	1	1	1	1	1
      | 1	1	1	1	1	1	0	0	0	0	0	0	0	1	1	1	1	1	1
      | 0	0	0	0	0	0	0	0	0	0	0	0	0	0	0	0	0	0	0
      | 0	0	0	0	0	0	0	0	0	0	0	0	0	0	0	0	0	0	0
      | 0	0	0	0	0	0	0	0	0	0	0	0	0	0	0	0	0	0	0
      | 0	0	0	0	0	0	0	0	0	0	0	0	0	0	0	0	0	0	0
      | 0	0	0	0	0	0	0	0	0	0	0	0	0	0	0	0	0	0	0
      | 0	0	0	0	0	0	0	0	0	0	0	0	0	0	0	0	0	0	0
      | 0	0	0	0	0	0	0	0	0	0	0	0	0	0	0	0	0	0	0
      | 1	1	1	1	1	1	0	0	0	0	0	0	0	1	1	1	1	1	1
      | 1	1	1	1	1	1	0	0	0	0	0	0	0	1	1	1	1	1	1
      | 1	1	1	1	1	1	0	0	0	0	0	0	0	1	1	1	1	1	1
      | 1	1	1	1	1	1	0	0	0	0	0	0	0	1	1	1	1	1	1
      | 1	1	1	1	1	1	0	0	0	0	0	0	0	1	1	1	1	1	1
      | 1	1	1	1	1	1	0	0	0	0	0	0	0	1	1	1	1	1	1]
  Triangle : Constant  Value=|  OutDataType=fixdt(1, 16)  OutScaling=2^0
      | [1	1	1	1	1	1	1	1	1	0	1	1	1	1	1	1	1	1	1
      | 1	1	1	1	1	1	1	1	1	0	1	1	1	1	1	1	1	1	1
      | 1	1	1	1	1	1	1	1	0	0	0	1	1	1	1	1	1	1	1
      | 1	1	1	1	1	1	1	1	0	0	0	1	1	1	1	1	1	1	1
      | 1	1	1	1	1	1	1	0	0	0	0	0	1	1	1	1	1	1	1
      | 1	1	1	1	1	1	1	0	0	0	0	0	1	1	1	1	1	1	1
      | 1	1	1	1	1	1	0	0	0	0	0	0	0	1	1	1	1	1	1
      | 1	1	1	1	1	1	0	0	0	0	0	0	0	1	1	1	1	1	1
      | 1	1	1	1	1	0	0	0	0	0	0	0	0	0	1	1	1	1	1
      | 1	1	1	1	1	0	0	0	0	0	0	0	0	0	1	1	1	1	1
      | 1	1	1	1	0	0	0	0	0	0	0	0	0	0	0	1	1	1	1
      | 1	1	1	1	0	0	0	0	0	0	0	0	0	0	0	1	1	1	1
      | 1	1	1	0	0	0	0	0	0	0	0	0	0	0	0	0	1	1	1
      | 1	1	1	0	0	0	0	0	0	0	0	0	0	0	0	0	1	1	1
      | 1	1	0	0	0	0	0	0	0	0	0	0	0	0	0	0	0	1	1
      | 1	1	0	0	0	0	0	0	0	0	0	0	0	0	0	0	0	1	1
      | 1	0	0	0	0	0	0	0	0	0	0	0	0	0	0	0	0	0	1
      | 1	0	0	0	0	0	0	0	0	0	0	0	0	0	0	0	0	0	1
      | 0	0	0	0	0	0	0	0	0	0	0	0	0	0	0	0	0	0	0]
  Templates : Outport  OutDataType=fixdt(1, 16)  OutScaling=2^0
  wires:
  Cruciform/1 -> Bus Creator/1  "Cruciform"
  Circle/1 -> Bus Creator/2  "Circle"
  Triangle/1 -> Bus Creator/3  "Triangle"
  Bus Creator/1 -> Templates/1

== system Lidar_System_FullState_Apr19_2015_Triangle/Enabled Subsystem1/Perception/Color Analysis/Template Matching (Docking)/Docking2/Recognition/Subsystem ==
  BBox in : Inport  OutDataType=fixdt(1, 16)  OutScaling=2^0
  Idx : Inport  Port=2  OutDataType=fixdt(1, 16)  OutScaling=2^0
  Permute Matrix : dspmtrx3/Permute Matrix  mode=Rows  ZeroOneIdxMode=One-based  errmode=Clip index  checkDims=off
  Sort : dspstat3/Sort  DialogController=dspDDGCreate  DialogControllerArgs=DataTag3  otype=Index  dir=Ascending  sortAlg=Quick sort  roundingMode=Floor  overflowMode=off
  Submatrix : dspmtrx3/Submatrix  RowSpan=One row  RowStartMode=First  RowStartIndex=1  RowEndMode=Index  RowEndIndex=3  ColSpan=All columns  ColStartMode=First  ColStartIndex=1  ColEndMode=Last  ColEndIndex=1
  BBox out : Outport  OutDataType=fixdt(1, 16)  OutScaling=2^0
  wires:
  Submatrix/1 -> BBox out/1
  Permute Matrix/1 -> Submatrix/1
  Sort/1 -> Permute Matrix/2
  BBox in/1 -> Permute Matrix/1
  Idx/1 -> Sort/1

== matlab function Enabled Subsystem1/Sensor Enable ==
  data: mode input double; choice output double
function choice = SEnab(mode)
% Input choice into S-Function
% Choice 0 - Lidar Only
% Choice 1 - Camera Only
% Choice 2 - Lidar and Camera

if (mode <= 5)
    choice = 2;
elseif (mode > 5)
    choice = 1;
else
    choice = 0;
end

end

== matlab function Enabled Subsystem1/Perception/Match Landmarks ==
  data: im_distances input double; idx output double; im_angles input double; Distances input double; Angles input double; distances output double; angles output double
function [idx, distances, angles] = MatchLandmarks(im_distances, im_angles, Distances, Angles)
%Written by Anderson Lebbad on August 9, 2014
%Last Edited:

%This function takes the distances and angles found from 'Color Analysis'
%and finds the index of that blob found in 'Detect Landmarks'

%Variable for the number of blobs that color analysis has been run on
num = 4;
idx = zeros(num,1);

distances = Distances;
angles = Angles;

% %Loop through each analysis blob
% for i = 1:num
%     %Check if a valid distance was found
%     if im_distances(i) ~= 0
%         %Calculate L1 norm to find how far the difference is for each
%         L1norm = abs(im_distances(i)-Distances) + abs(im_angles(i)-Angles);
%         %find the minimum
%         [C,I] = min(L1norm);
%         %record the index
%         idx(i) = I(1);
%     else
%         %Invalid distance (no object found)
%         idx(i) = 0;
%     end
% end

if im_distances(1) ~= 0
    distances(9:12) = im_distances;
    angles(9:12) = im_angles;
    idx = (9:12)'.*(im_distances ~= 0);
end

end

== matlab function Enabled Subsystem1/Perception/Raster to UV scatter1 ==
  data: scanAngle output double; gimbalAngle output double; range output double; DistIM input double
function [ scanAngle, gimbalAngle, range ] = imageToPoints( DistIM )
%Written by Anderson Lebbad on August 27, 2014
%Last Edited:

%This function takes a depth image as saved from the pandaboard and back
%propagates a list of points to be used for the mapper

highAngle = 10;
lowAngle = -35;

rows = 65;
cols = 540;
SAmat = zeros(rows,cols);
GAmat = zeros(rows,cols);
scanAngle = zeros(rows*cols,1);
gimbalAngle = zeros(rows*cols,1);
range = zeros(rows*cols,1);

for i=1:rows
    SAmat(i,:) = 157.25:-.25:22.5;
    GAmat(i,:) = highAngle-(i-1)*(highAngle-lowAngle)/(rows-1);
end

range(:) = DistIM';
scanAngle(:) = SAmat';
gimbalAngle(:) = GAmat';

end

== matlab function Enabled Subsystem1/Perception/Detect Landmarks/Embedded MATLAB Function1 ==
  data: centroid input double; bbox input double; BW input double; dist_im input double; Distances output double; Angles output double
function [Distances, Angles] = landmarkInfo(centroid, bbox, BW, dist_im)
%Written by Anderson Lebbad on July 22, 2014
%Last Edited:

%This function finds the average depth of a detected blob and the relative
%angle of it

%Initialize variables
numBlobs = 12;
Distances = zeros(1,numBlobs);
Angles = zeros(1,numBlobs);

for k=1:numBlobs
    %Initialize loop variables
    pixels = 0;
    DRunAve = 0;
    angleCalc = 0;
    
    %Parse bbox data for the current blob
    left = bbox(2,k) + 1;
    right = left + bbox(4,k) - 1;
    bottom = bbox(1,k) + 1;
    top = bottom + bbox(3,k) - 1;
    
    
    
    %Check to see if valid bbox is found
    if left~=0
        %Calculate angle based off centroid. Dist_im has 540 horizontal columns
        %that cover a 135 field of view (4 points per degree)
        angleCalc = centroid(2,k)/4 - 67.5;
        %Scan the detected region of the binary image and generate histograms
        for j=left:right
            for i=bottom:top
                if BW(i,j) == 1
                    pixels = pixels + 1;
                    DRunAve = ((pixels-1)/pixels)*DRunAve + (1/pixels)*double(dist_im(i,j));
                end
            end
        end
    end
    
    %Output distance in cm
    Distances(k) = round(DRunAve/10);
    %Output angle as a positive integer
    Angles(k) = mod(round(angleCalc),360);
    
end

end

== matlab function Enabled Subsystem1/Perception/Raster to UV scatter ==
  data: depthImage output double; scanAngle input double; gimbalAngle input double; range input double; upScan input double
function depthImage  = lidarMapper( scanAngle, gimbalAngle, range, upScan )
%Written by Anderson Lebbad on July 30, 2014
%Last Edited: September 6, 2014 for reduction to valid points

%This function takes the lidar data and transforms it to pixel coordinates
%in the image frame, then maps the depths to a 'depth image' to be used for
%fusion based analysis (specifically color estimation)

% %% Reduce to only points with valid data
% valid = (range > 0) & (range < 30000);
% validIdx = (1:length(valid))'.*valid;
% numValid = sum(valid);
% validIdx = sort(validIdx,'descend');
% validIdx = validIdx(1:numValid);
% range = range(validIdx);
% gimbalAngle = gimbalAngle(validIdx);
% scanAngle = scanAngle(validIdx);

%% Convert angles to radians
scanAngleR = scanAngle*pi/180;
gimbalAngleR = gimbalAngle*pi/180;

%% Initialize matrix sizes for operation
depthImage = zeros(480,640);

%% System Parameters

% Height of the lidar on the gimbal
h = 36.3;

% Translation vector (in centimeters)
t = [2.4; -11.3; 3.8];
% Rotation angles
phi = (-90-12.5)*pi/180;
theta = 2.5*pi/180;
if upScan == 1
    phi = (-90-0.5)*pi/180;
end
    
% Rotation about the x-axis
Rx = [1 0 0; 0 cos(phi) sin(phi); 0 -sin(phi) cos(phi)];
% Followed by rotation about the y-axis
R = [cos(theta) 0 -sin(theta); 0 1 0; sin(theta) 0 cos(theta)]*Rx;
% Transformation matrix
T = [R t];

% Radial Distortions
RadDist = [0.069102182282360,-0.154608606024690,0.020241053576861];

% Intrinsic Matrix
K = [5.548581600685270e+02,0,0;0,5.523116000564020e+02,0;3.135858904821101e+02,2.190392333699872e+02,1];
KK = K';

%% Get pixel values

% Convert to XYZ
X = range.*cos(scanAngleR);
Y = range.*sin(scanAngleR).*cos(gimbalAngleR)-h.*sin(gimbalAngleR);
Z = range.*sin(scanAngleR).*sin(gimbalAngleR)+h.*cos(gimbalAngleR);

% Transformation to camera coordinate frame
Xc = T(1,1).*X+T(1,2).*Y+T(1,3).*Z+T(1,4);
Yc = T(2,1).*X+T(2,2).*Y+T(2,3).*Z+T(2,4);
Zc = T(3,1).*X+T(3,2).*Y+T(3,3).*Z+T(3,4);

% Normalize Coordinates
Xn = Xc./Zc;
Yn = Yc./Zc;

% Calculate Distance to each point from camera
Dp = sqrt(Xc.^2+Yc.^2+Zc.^2);

% Radial Vectors
r2 = Xn.^2+Yn.^2;
r6 = r2.^3;

% Distorted Coordinates
Xd = Xn.*(1+RadDist(1).*r2+RadDist(3).*r6);
Yd = Yn.*(1+RadDist(1).*r2+RadDist(3).*r6);

% Pixel Coordinates
Xp = KK(1,1).*Xd+KK(1,2).*Yd+KK(1,3);
Yp = KK(2,1).*Xd+KK(2,2).*Yd+KK(2,3);

%% Create sparse distance array

for k=1:length(Xp)
    xi = round(Xp(k));
    yi = round(Yp(k));
    if xi>0 && xi<=640 && yi>0 && yi<=480
        if depthImage(yi,xi) == 0
            depthImage(yi,xi) = Dp(k);
        else
            depthImage(yi,xi) = (depthImage(yi,xi)+Dp(k))/2;
        end
    end
end

end

== matlab function Enabled Subsystem1/Perception/Color Analysis/Find Can Buoys/Embedded MATLAB Function1 ==
  data: centroid input double; bbox input double; BW input double; dist_im input double; Distances output double; Angles output double
function [Distances, Angles] = landmarkInfo(centroid, bbox, BW, dist_im)
%Written by Anderson Lebbad on July 22, 2014
%Last Edited:

%This function finds the average depth of a detected blob and the relative
%angle of it

%Initialize variables
numBlobs = 4;
Distances = zeros(4,1);
Angles = zeros(4,1);

for k=1:numBlobs
    %Initialize loop variables
    pixels = 0;
    DRunAve = 0;
    angleCalc = 0;
    
    %Parse bbox data for the current blob
    left = bbox(2,k) + 1;
    right = left + bbox(4,k) - 1;
    bottom = bbox(1,k) + 1;
    top = bottom + bbox(3,k) - 1;
    
    
    
    %Check to see if valid bbox is found
    if left~=0
        %Calculate angle based off centroid. Dist_im has 540 horizontal columns
        %that cover a 135 field of view (4 points per degree)
        angleCalc = centroid(2,k)/4 - 67.5;
        %Scan the detected region of the binary image and generate histograms
        for j=left:right
            for i=bottom:top
                if BW(i,j) == 1
                    pixels = pixels + 1;
                    DRunAve = ((pixels-1)/pixels)*DRunAve + (1/pixels)*double(dist_im(i,j));
                end
            end
        end
    end
    
    %Output distance in cm
    Distances(k) = round(DRunAve/10);
    %Output angle as a positive integer
    Angles(k) = mod(round(angleCalc),360);
    
end

end

== matlab function Enabled Subsystem1/Perception/Color Analysis/Template Matching (Docking)/Docking2/Blob Analysis/BBox Transform ==
  data: BBin input double; BBout output double
function BBout = Btrans(BBin)
%Change BBbox from 2009 layout to 2014 layout to work with other code

BBinT = BBin';

x1 = BBinT(:,2);
y1 = BBinT(:,1);
h1 = BBinT(:,3);
w1 = BBinT(:,4);

BBout = [x1 y1 w1 h1];

== matlab function Enabled Subsystem1/Perception/Color Analysis/Template Matching (Docking)/Docking2/Detection/Detection ==
  data: cruciform input double; bbox_out output double; circle input double; triangle input double; whitePixCount input double; threshold input double; V_mask input double; bbox_in input double; label input double; rtnRatioDiff output double
function [bbox_out,rtnRatioDiff]= detection(cruciform,circle,triangle,...
    whitePixCount,threshold,V_mask,bbox_in,label)

% Written by Edward Zhu on 5/14/14

% Inputs
% tempID:       Number corresponding to one of the templates (cruciform: 1,
%               circle: 2, triangle: 3)
% cruciform:    19*19 template of cruciform
% circle:       19*19 template of circle
% triangle:     19*19 template of triangle
% whitePixCount:Number of white pixels in each of the templates
% V_mask:       V channel binary mask
% bbox_in:      Bounding boxes as found by blob analysis
% label:        Label matrix as found by blob analysis

% Outputs
% bbox_out:     Bounding box of matched symbol
% symFound:     Status of matching (found: 1, not found: 0)

% Define frame and template size
templates = zeros(19,19,3);
templates(:,:,1) = cruciform;
templates(:,:,2) = circle;
templates(:,:,3) = triangle;

imgRows = size(label,1);
imgCols = size(label,2);
tempRows = size(templates,1);
tempCols = size(templates,2);
numBBox = size(bbox_in,1);

% Initialize scaled image and output bbox matrices
V_scaled = zeros(tempRows,tempCols);
bbox_out = uint32(zeros(numBBox,4));
rtnRatioDiff = ones(numBBox,1);

bestRatioDiff = single(1);

for i = 1:numBBox
    shapeDiff = abs(1-bbox_in(i,3)/bbox_in(i,4));
    if bbox_in(i,3) >= tempCols && bbox_in(i,4) >= tempRows && shapeDiff < 0.5
        % Set up arrays for the start and end rows and columns for bbox
        % matching
        
        similarity = zeros(1,3);
        ratioDiff = zeros(1,3);
        
        rowStep = floor(bbox_in(i,4) / tempRows);
        colStep = floor(bbox_in(i,3) / tempCols);
        
        startRowList = zeros(1,3);
        startRowList(2) = bbox_in(i,2);
        startRowList(1) = max(1, startRowList(2) - rowStep);
        startRowList(3) = min(imgRows, startRowList(2) + rowStep);
        
        endRowList = zeros(1,3);
        endRowList(2) = bbox_in(i,2) + bbox_in(i,4);
        endRowList(1) = max(1, endRowList(2) - rowStep);
        endRowList(3) = min(imgRows, endRowList(2) + rowStep);
        
        startColList = zeros(1,3);
        startColList(2) = bbox_in(i,1);
        startColList(1) = max(1, startColList(2) - colStep);
        startColList(3) = min(imgCols, startColList(2) + colStep);
        
        endColList = zeros(1,3);
        endColList(2) = bbox_in(i,1) + bbox_in(i,3);
        endColList(1) = max(1, endColList(2) - colStep);
        endColList(3) = min(imgCols, endColList(2) + colStep);
        
        % Scale down image in bbox to size of template (18*18 px)
        for startRow = startRowList
            for endRow = endRowList
                rowScaleStep = floor((endRow - startRow) / tempRows);
                
                for startCol = startColList
                    for endCol = endColList
                        colScaleStep = floor((endCol - startCol) / tempCols);
                        
                        captureRow = startRow;
                        for row = 1:tempRows
                            captureCol = startCol;
                            for col = 1:tempCols
                                V_scaled(row,col) = V_mask(captureRow,captureCol);
                                for tempID = 1:3
                                    similarity(tempID) = similarity(tempID) + templates(row,col,tempID) * (V_mask(captureRow,captureCol)*(-1) + 1);
                                end
                                captureCol = captureCol + colScaleStep;                        
                            end
                            captureRow = captureRow + rowScaleStep;
                        end                  
                        
                        for tempID = 1:3   
                            ratioDiff(tempID) = abs(1 - single(similarity(tempID)) / single(whitePixCount(tempID))); 
                        end
                        
                        if min(ratioDiff) < bestRatioDiff
                            bestRatioDiff = single(min(ratioDiff));
                        end
                    end
                end
            end
        end
        
        % Output valid bounding boxes
        if bestRatioDiff < threshold
            bbox_out(i,:) = bbox_in(i,:);
            rtnRatioDiff(i) = bestRatioDiff;
        end
    end
end

== matlab function Enabled Subsystem1/Perception/Color Analysis/Template Matching (Docking)/Docking2/Embedded MATLAB Function ==
  data: xRec input double; bayNumber output double; xDet input double
function bayNumber = bayPosition(xRec,xDet)

symxpos = xRec(1);

diff1 = xDet(1) - symxpos;
diff2 = xDet(2) - symxpos;
diff3 = xDet(3) - symxpos;

if diff1 == 0
    bayNumber = uint8(1);
elseif diff2 == 0
    bayNumber = uint8(2);
elseif diff3 == 0
    bayNumber = uint8(3);
else
    bayNumber = uint8(0);
end

== matlab function Enabled Subsystem1/Perception/Raster Image ==
  data: lidarData input double; dist_image output double; UpDown input double
function dist_image = scanImages(lidarData,UpDown)
%Written by Anderson Lebbad on July 5, 2014
%Last Edited:

%Converts the one dimensional array of lidarData and the scan settings into
%frames of distances and angles for each point

% Set output sizes
dist_image = zeros(65,540);

% To run through the middle half of the points horizonatal points, the
% first quarter must be skipped (of 1080)
scanOffset = 270-1;

% Loop through all points in output matrices
for j=1:540
    for i=1:65
        % Select the lidarData that will be used in analysis and format as
        % a frame
        dist_image(i,j) = lidarData(j+scanOffset+1080*(i-1));
    end
end

% Flip if up scan
if UpDown
    dist_image = flipud(dist_image);
end

dist_image = fliplr(dist_image);

end

== matlab function Enabled Subsystem1/Perception/Lidar data selector ==
  data: lidarIn input double; lidarOut output double
function lidarOut = data_selector(lidarIn)
% Lidar data is always input as a 1x70200 matrix.
% If Scan Number is less than 65 some of this data may be blank
% Select only the parts of the matrix where data has been collected

FullLength = 1080*65;
DataLength =  1080*65;
lidarOut = zeros(FullLength,1);

% ClosePts = (lidarIn < 3);
% lidarOut = (lidarIn + 30000*ClosePts)/10;

for i = 1:DataLength
    if (lidarIn(i,1) < 3)
        lidarIn(i,1) = 30000;
    end
    lidarOut(i,1) = lidarIn(i,1);
end

%lidarOut = lidarIn(1,1:DataLength);
